simulink model "gm_signalSim"  (R2023b)
settings: Solver=VariableStepAuto  StartTime=0.0  StopTime=0.001  RelTol=1e-3
undefined symbols (not defined in the file or in its folder): f, fdac, fs, inc_1e5
libraries: hdlsllib x5, dspsrcs4 x4, dspfdesign x2, dsphdlsigops2 x1
settings Model: Creator=31651  LastModifiedBy=31651
settings OptimizationCC: BlockReduction=off  ConditionallyExecuteInputs=off
settings DebuggingCC: InheritedTsInSrcMsg=none

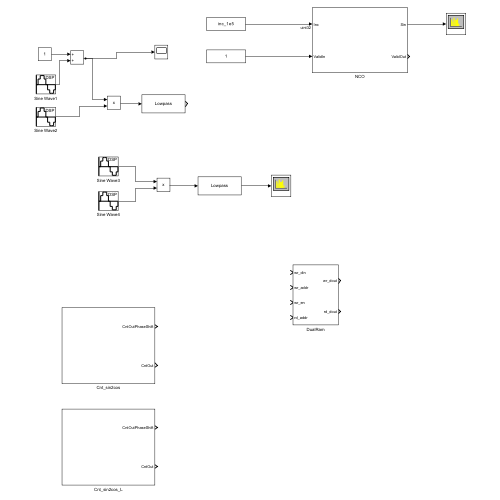
[thumbnail: Simulink's stored preview of the top-level diagram]
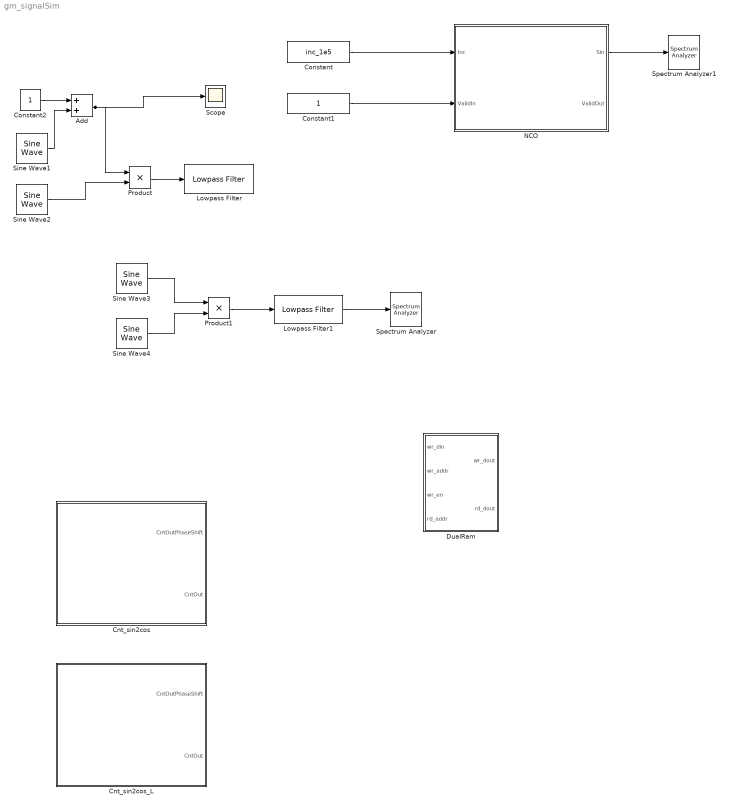
== system gm_signalSim ==
  Add : Sum
  Cnt_sin2cos : Subsystem
  Cnt_sin2cos_L : Subsystem
  Constant : Constant  Value=inc_1e5  OutDataTypeStr=uint32  SampleTime=1/fdac
  Constant1 : Constant  OutDataTypeStr=boolean  SampleTime=1/fdac
  Constant2 : Constant  SampleTime=1/fs
  DualRam : Subsystem
  Lowpass Filter : dspfdesign/Lowpass Filter  FilterType=FIR  DesignForMinimumOrder=on  FilterOrder=50  PassbandFrequency=500  StopbandFrequency=1500  PassbandRipple=0.1  StopbandAttenuation=80  SampleRateMode=Specify on dialog  SampleRate=fs  SimulateUsing=Interpreted execution  roundingMode=Floor  coeffsDataTypeStr=fixdt(1,16)
  Lowpass Filter1 : dspfdesign/Lowpass Filter  FilterType=FIR  DesignForMinimumOrder=on  FilterOrder=50  PassbandFrequency=500  StopbandFrequency=1500  PassbandRipple=0.1  StopbandAttenuation=80  SampleRateMode=Specify on dialog  SampleRate=fs  SimulateUsing=Interpreted execution  roundingMode=Floor  coeffsDataTypeStr=fixdt(1,16)
  NCO : Subsystem
  Product : Product
  Product1 : Product
  Scope : Scope
  Sine Wave1 : dspsrcs4/Sine Wave  Amplitude=1  Frequency=f  Phase=pi/2  SampleMode=Discrete  OutComplex=Real  CompMethod=Trigonometric fcn  TableSize=Speed  SampleTime=1/fs  SamplesPerFrame=1  ResetState=Restart at time zero  OutputFrames=off  dataType=double  wordLen=16  udDataType=sfix(16)  fracBitsMode=Best precision  numFracBits=15  OutDataTypeStr=double  LastOutDataTypeStr=double
  Sine Wave2 : dspsrcs4/Sine Wave  Amplitude=1  Frequency=f  Phase=-pi/6  SampleMode=Discrete  OutComplex=Real  CompMethod=Trigonometric fcn  TableSize=Speed  SampleTime=1/fs  SamplesPerFrame=1  ResetState=Restart at time zero  OutputFrames=off  dataType=double  wordLen=16  udDataType=sfix(16)  fracBitsMode=Best precision  numFracBits=15  OutDataTypeStr=double  LastOutDataTypeStr=double
  Sine Wave3 : dspsrcs4/Sine Wave  Amplitude=1  Frequency=f  Phase=0  SampleMode=Discrete  OutComplex=Real  CompMethod=Trigonometric fcn  TableSize=Speed  SampleTime=1/fs  SamplesPerFrame=1  ResetState=Restart at time zero  OutputFrames=off  dataType=double  wordLen=16  udDataType=sfix(16)  fracBitsMode=Best precision  numFracBits=15  OutDataTypeStr=double  LastOutDataTypeStr=double
  Sine Wave4 : dspsrcs4/Sine Wave  Amplitude=1  Frequency=f  Phase=0  SampleMode=Discrete  OutComplex=Real  CompMethod=Trigonometric fcn  TableSize=Speed  SampleTime=1/fs  SamplesPerFrame=1  ResetState=Restart at time zero  OutputFrames=off  dataType=double  wordLen=16  udDataType=sfix(16)  fracBitsMode=Best precision  numFracBits=15  OutDataTypeStr=double  LastOutDataTypeStr=double
  Spectrum Analyzer : SpectrumAnalyzer  WindowPosition=[450.000000,323.000000,800.000000,500.000000,]  Visible=on  ScopeFrameLocation=window  Span=1000000  StartFrequency=-500000  StopFrequency=500000  YLimits=[-255.53959036,54.82932114]
  Spectrum Analyzer1 : SpectrumAnalyzer  WindowPosition=[264.000000,231.000000,800.000000,500.000000,]  Visible=on  ScopeFrameLocation=window  YLimits=[-124.62359501,39.65782076]  SelectedToolstripTab=spectrumAnalyzerToolstrip.measurementsTab
  wires:
  Lowpass Filter1/1 -> Spectrum Analyzer/1
  Product1/1 -> Lowpass Filter1/1
  Sine Wave4/1 -> Product1/2
  Sine Wave3/1 -> Product1/1
  Add/1 -> Product/1, Scope/1
  Sine Wave1/1 -> Add/2
  Constant2/1 -> Add/1
  Constant/1 -> NCO/1(Inc)
  NCO/1(Sin) -> Spectrum Analyzer1/1
  Constant1/1 -> NCO/2(ValidIn)
  Product/1 -> Lowpass Filter/1
  Sine Wave2/1 -> Product/2

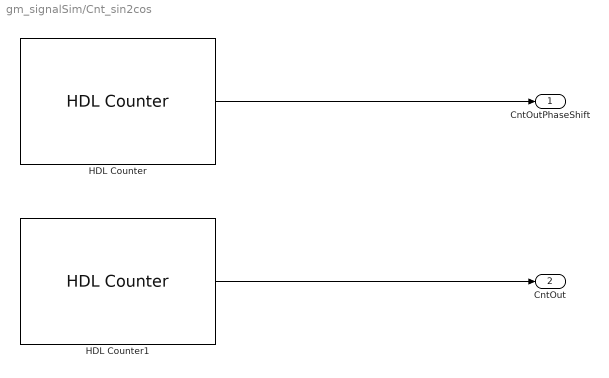
== system gm_signalSim/Cnt_sin2cos ==
  HDL Counter : hdlsllib/Sources/HDL Counter  CountType=Count limited  CountInit=50  CountStep=1  CountMax=1000  CountFromType=Specify  CountFrom=1  CountResetPort=off  CountLoadPort=off  CountEnbPort=off  CountDirPort=off  CountHitOutputPort=off  CountDataType=Unsigned  CountWordLen=10  CountFracLen=0  CountSampTime=1/fs
  HDL Counter1 : hdlsllib/Sources/HDL Counter  CountType=Count limited  CountInit=1  CountStep=1  CountMax=1000  CountFromType=Specify  CountFrom=1  CountResetPort=off  CountLoadPort=off  CountEnbPort=off  CountDirPort=off  CountHitOutputPort=off  CountDataType=Unsigned  CountWordLen=10  CountFracLen=0  CountSampTime=1/fs
  CntOutPhaseShift : Outport  VectorParamsAs1DForOutWhenUnconnected=off
  CntOut : Outport  Port=2  VectorParamsAs1DForOutWhenUnconnected=off
  wires:
  HDL Counter1/1 -> CntOut/1
  HDL Counter/1 -> CntOutPhaseShift/1

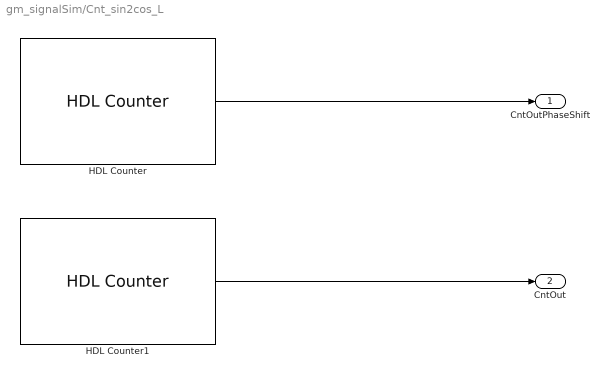
== system gm_signalSim/Cnt_sin2cos_L ==
  HDL Counter : hdlsllib/Sources/HDL Counter  CountType=Count limited  CountInit=5  CountStep=1  CountMax=1000  CountFromType=Specify  CountFrom=1  CountResetPort=off  CountLoadPort=off  CountEnbPort=off  CountDirPort=off  CountHitOutputPort=off  CountDataType=Unsigned  CountWordLen=10  CountFracLen=0  CountSampTime=1/fs
  HDL Counter1 : hdlsllib/Sources/HDL Counter  CountType=Count limited  CountInit=1  CountStep=1  CountMax=1000  CountFromType=Specify  CountFrom=1  CountResetPort=off  CountLoadPort=off  CountEnbPort=off  CountDirPort=off  CountHitOutputPort=off  CountDataType=Unsigned  CountWordLen=10  CountFracLen=0  CountSampTime=1/fs
  CntOutPhaseShift : Outport  VectorParamsAs1DForOutWhenUnconnected=off
  CntOut : Outport  Port=2  VectorParamsAs1DForOutWhenUnconnected=off
  wires:
  HDL Counter/1 -> CntOutPhaseShift/1
  HDL Counter1/1 -> CntOut/1

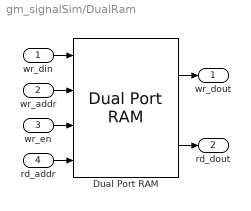
== system gm_signalSim/DualRam ==
  wr_din : Inport  OutDataTypeStr=uint8
  wr_addr : Inport  Port=2
  wr_en : Inport  Port=3
  rd_addr : Inport  Port=4
  Dual Port RAM : hdlsllib/HDL RAMs/Dual Port RAM  ram_size=10
  wr_dout : Outport
  rd_dout : Outport  Port=2
  wires:
  wr_en/1 -> Dual Port RAM/3
  Dual Port RAM/1 -> wr_dout/1
  wr_din/1 -> Dual Port RAM/1
  wr_addr/1 -> Dual Port RAM/2
  Dual Port RAM/2 -> rd_dout/1
  rd_addr/1 -> Dual Port RAM/4

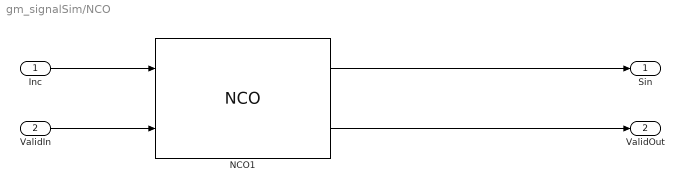
== system gm_signalSim/NCO ==
  Inc : Inport  OutDataTypeStr=uint32
  ValidIn : Inport  Port=2
  NCO1 : dsphdlsigops2/NCO  PhaseIncrementSource=Input port  PhaseIncrement=inc_1e5  PhaseOffsetSource=Property  PhaseOffset=0  DitherSource=Property  NumDitherBits=4  SamplesPerFrame=1  LUTCompress=off  ResetAction=off  Waveform=Sine  PhasePort=off  SimulateUsing=Code generation  AccumulatorWL=N  PhaseQuantization=on  NumQuantizerAccumulatorBits=12  OutputDataType=Binary point scaling  OutputWL=12  OutputFL=10
  Sin : Outport
  ValidOut : Outport  Port=2
  wires:
  NCO1/1 -> Sin/1
  ValidIn/1 -> NCO1/2
  Inc/1 -> NCO1/1
  NCO1/2 -> ValidOut/1
